simulink model "mpc_con_2018"  (R2018a)
settings: Solver=VariableStepAuto  StartTime=0.0  StopTime=time_end  RelTol=1e-3
values from neighbouring files (symbols this model uses):
  h_01 = 10.17    [script_mpc_con.m]
  h_02 = 10.53    [script_mpc_con.m]
  Td = 0.5    [script_mpc_con.m]
  u_max = repmat(u_max,Nc,1)    [script_mpc_con.m]
  u_min = repmat(u_min,Nc,1)    [script_mpc_con.m]
  ue = [ue1; ue2]    [script_mpc_con.m]
  x_max = repmat(x_max,Np,1)    [script_mpc_con.m]
  x_min = repmat(x_min,Np,1)    [script_mpc_con.m]
  xe = [xe1; xe2]    [script_mpc_con.m]
  xe1 = (k_2*sqrt(xe2)/k_1)^2    [script_mpc_con.m]
  xe2 = 25.53    [script_mpc_con.m]
undefined symbols (not defined in the file or in its folder): A, B, C, Fx, Fy, Gx, Gy
settings Model: Creator=NicSch02  LastModifiedBy=NicSch02
settings DataIOCC: ReturnWorkspaceOutputs=on
settings SFSimCC: SimUseLocalCustomCode=on
settings RTWCC: RTWUseLocalCustomCode=on

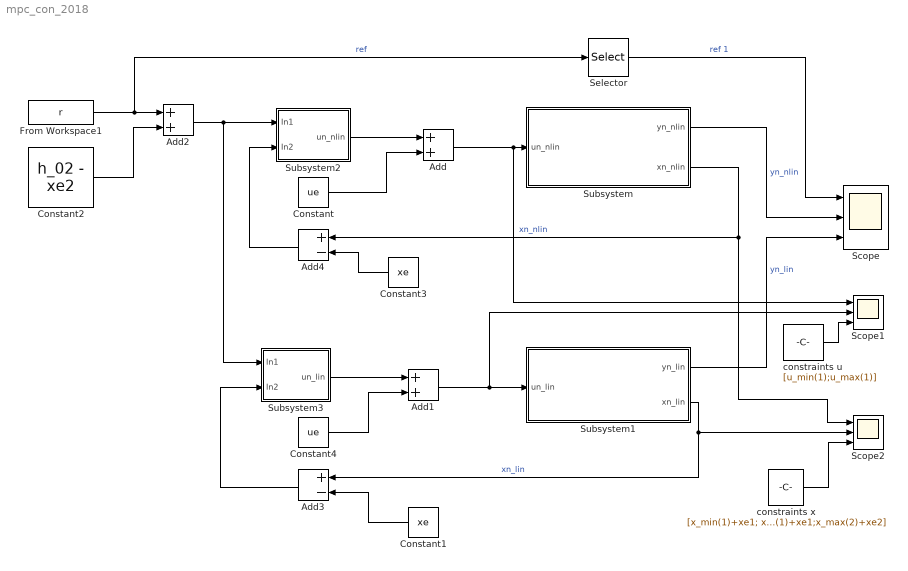
== system mpc_con_2018 ==
  Add : Sum
  Add1 : Sum
  Add2 : Sum
  Add3 : Sum  Inputs=+-
  Add4 : Sum  Inputs=+-
  Constant : Constant  Value=ue
  Constant1 : Constant  Value=xe
  Constant2 : Constant  Value=h_02 - xe2
  Constant3 : Constant  Value=xe
  Constant4 : Constant  Value=ue
  From Workspace1 : FromWorkspace  VariableName=r  SampleTime=0
  Scope : Scope  NumInputPorts=3
  Scope1 : Scope  NumInputPorts=3
  Scope2 : Scope  NumInputPorts=3
  Selector : Selector  InputPortWidth=Np  IndexOptions=Index vector (dialog)  Indices=[1]  OutputSizes=1
  Subsystem : Subsystem
  Subsystem1 : Subsystem
  Subsystem2 : Subsystem
  Subsystem3 : Subsystem
  constraints u : Constant  Value=[u_min(1);u_max(1)]
  constraints x : Constant  Value=[x_min(1)+xe1; x_min(2)+xe2; x_max(1)+xe1;x_max(2)+xe2]
  wires:
  Subsystem/1(yn_nlin) -> Scope/2  "yn_nlin"
  Subsystem1/1(yn_lin) -> Scope/3  "yn_lin"
  Subsystem/2(xn_nlin) -> Scope2/1, Add4/1  "xn_nlin"
  Subsystem1/2(xn_lin) -> Add3/1, Scope2/2  "xn_lin"
  Selector/1 -> Scope/1  "ref 1"
  Constant2/1 -> Add2/2
  From Workspace1/1 -> Selector/1, Add2/1  "ref"
  Add2/1 -> Subsystem3/1(In1), Subsystem2/1(In1)
  constraints x/1 -> Scope2/3
  constraints u/1 -> Scope1/3
  Constant1/1 -> Add3/2
  Constant3/1 -> Add4/2
  Add/1 -> Scope1/1, Subsystem/1(un_nlin)
  Constant/1 -> Add/2
  Add4/1 -> Subsystem2/2(In2)
  Subsystem2/1(un_nlin) -> Add/1
  Add1/1 -> Subsystem1/1(un_lin), Scope1/2
  Constant4/1 -> Add1/2
  Add3/1 -> Subsystem3/2(In2)
  Subsystem3/1(un_lin) -> Add1/1

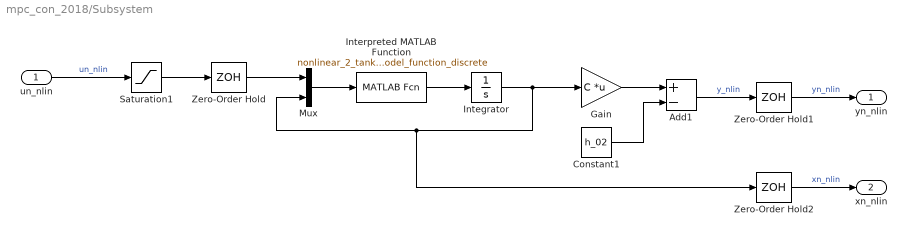
== system mpc_con_2018/Subsystem ==
  un_nlin : Inport
  Add1 : Sum  Inputs=+-
  Constant1 : Constant  Value=h_02
  Gain : Gain  Gain=C  Multiplication=Matrix(K*u)
  Integrator : Integrator  InitialCondition=[h_01;h_02]
  Interpreted MATLAB Function : MATLABFcn  MATLABFcn=nonlinear_2_tank_model_function_discrete
  Mux : Mux  Inputs=2
  Saturation1 : Saturate  UpperLimit=u_max(1)  LowerLimit=u_min(1)
  Zero-Order Hold : ZeroOrderHold  SampleTime=Td
  Zero-Order Hold1 : ZeroOrderHold  SampleTime=Td
  Zero-Order Hold2 : ZeroOrderHold  SampleTime=Td
  yn_nlin : Outport
  xn_nlin : Outport  Port=2
  wires:
  Integrator/1 -> Zero-Order Hold2/1, Mux/2, Gain/1
  Constant1/1 -> Add1/2
  Interpreted MATLAB Function/1 -> Integrator/1
  Gain/1 -> Add1/1
  Mux/1 -> Interpreted MATLAB Function/1
  un_nlin/1 -> Saturation1/1  "un_nlin"
  Zero-Order Hold/1 -> Mux/1
  Add1/1 -> Zero-Order Hold1/1  "y_nlin"
  Zero-Order Hold1/1 -> yn_nlin/1  "yn_nlin"
  Saturation1/1 -> Zero-Order Hold/1
  Zero-Order Hold2/1 -> xn_nlin/1  "xn_nlin"

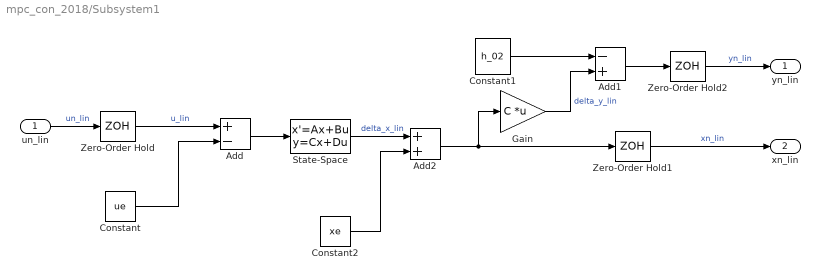
== system mpc_con_2018/Subsystem1 ==
  un_lin : Inport
  Add : Sum  Inputs=+-
  Add1 : Sum  Inputs=-+
  Add2 : Sum
  Constant : Constant  Value=ue
  Constant1 : Constant  Value=h_02
  Constant2 : Constant  Value=xe
  Gain : Gain  Gain=C  Multiplication=Matrix(K*u)
  State-Space : StateSpace  A=A  B=B  C=[[1,0];[0,1]]  D=[[0,0];[0,0]]  InitialCondition=[h_01;h_02] - xe
  Zero-Order Hold : ZeroOrderHold  SampleTime=Td
  Zero-Order Hold1 : ZeroOrderHold  SampleTime=Td
  Zero-Order Hold2 : ZeroOrderHold  SampleTime=Td
  yn_lin : Outport
  xn_lin : Outport  Port=2
  wires:
  un_lin/1 -> Zero-Order Hold/1  "un_lin"
  Zero-Order Hold1/1 -> xn_lin/1  "xn_lin"
  Zero-Order Hold2/1 -> yn_lin/1  "yn_lin"
  Add1/1 -> Zero-Order Hold2/1
  Constant1/1 -> Add1/1
  Gain/1 -> Add1/2  "delta_y_lin"
  Add/1 -> State-Space/1
  Zero-Order Hold/1 -> Add/1  "u_lin"
  Constant/1 -> Add/2
  State-Space/1 -> Add2/1  "delta_x_lin"
  Add2/1 -> Gain/1, Zero-Order Hold1/1
  Constant2/1 -> Add2/2

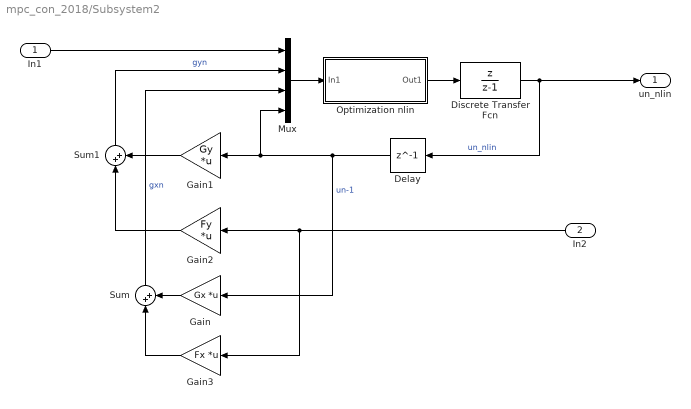
== system mpc_con_2018/Subsystem2 ==
  In1 : Inport
  In2 : Inport  Port=2
  Delay : Delay  DelayLength=1  InitialCondition=[0;0]  SampleTime=Td
  Discrete Transfer Fcn : DiscreteTransferFcn  Numerator=[1 0]  Denominator=[1 -1]  InitialStates=[0;0]  SampleTime=Td
  Gain : Gain  Gain=Gx  Multiplication=Matrix(K*u)
  Gain1 : Gain  Gain=Gy  Multiplication=Matrix(K*u)
  Gain2 : Gain  Gain=Fy  Multiplication=Matrix(K*u)
  Gain3 : Gain  Gain=Fx  Multiplication=Matrix(K*u)
  Mux : Mux
  Optimization nlin : Subsystem  TreatAsAtomicUnit=on  SystemSampleTime=Td
  Sum : Sum  Inputs=|++
  Sum1 : Sum  Inputs=|++
  un_nlin : Outport
  wires:
  Gain2/1 -> Sum1/1
  Gain1/1 -> Sum1/2
  Delay/1 -> Gain/1, Mux/4, Gain1/1  "un-1"
  Gain3/1 -> Sum/1
  Mux/1 -> Optimization nlin/1(In1)
  In2/1 -> Gain3/1, Gain2/1
  Discrete Transfer Fcn/1 -> un_nlin/1, Delay/1  "un_nlin"
  Gain/1 -> Sum/2
  Optimization nlin/1(Out1) -> Discrete Transfer Fcn/1
  Sum/1 -> Mux/3  "gxn"
  Sum1/1 -> Mux/2  "gyn"
  In1/1 -> Mux/1

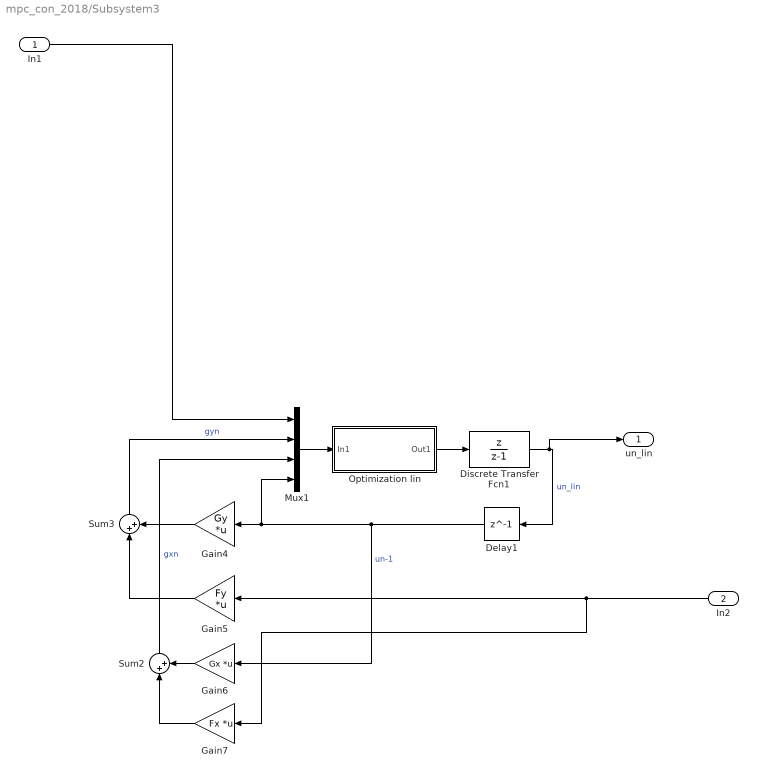
== system mpc_con_2018/Subsystem3 ==
  In1 : Inport
  In2 : Inport  Port=2
  Delay1 : Delay  DelayLength=1  InitialCondition=[0;0]  SampleTime=Td
  Discrete Transfer Fcn1 : DiscreteTransferFcn  Numerator=[1 0]  Denominator=[1 -1]  InitialStates=[0;0]  SampleTime=Td
  Gain4 : Gain  Gain=Gy  Multiplication=Matrix(K*u)
  Gain5 : Gain  Gain=Fy  Multiplication=Matrix(K*u)
  Gain6 : Gain  Gain=Gx  Multiplication=Matrix(K*u)
  Gain7 : Gain  Gain=Fx  Multiplication=Matrix(K*u)
  Mux1 : Mux
  Optimization lin : Subsystem  TreatAsAtomicUnit=on  SystemSampleTime=Td
  Sum2 : Sum  Inputs=|++
  Sum3 : Sum  Inputs=|++
  un_lin : Outport
  wires:
  Delay1/1 -> Gain6/1, Mux1/4, Gain4/1  "un-1"
  Sum3/1 -> Mux1/2  "gyn"
  Gain5/1 -> Sum3/1
  Gain4/1 -> Sum3/2
  Gain7/1 -> Sum2/1
  Discrete Transfer Fcn1/1 -> un_lin/1, Delay1/1  "un_lin"
  In2/1 -> Gain5/1, Gain7/1
  Optimization lin/1(Out1) -> Discrete Transfer Fcn1/1
  Sum2/1 -> Mux1/3  "gxn"
  Mux1/1 -> Optimization lin/1(In1)
  Gain6/1 -> Sum2/2
  In1/1 -> Mux1/1

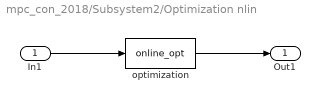
== system mpc_con_2018/Subsystem2/Optimization nlin ==
  In1 : Inport
  optimization : MATLABFcn  MATLABFcn=online_opt
  Out1 : Outport
  wires:
  In1/1 -> optimization/1
  optimization/1 -> Out1/1

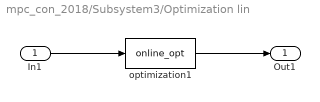
== system mpc_con_2018/Subsystem3/Optimization lin ==
  In1 : Inport
  optimization1 : MATLABFcn  MATLABFcn=online_opt
  Out1 : Outport
  wires:
  In1/1 -> optimization1/1
  optimization1/1 -> Out1/1
